simulink model "testVisualizer2023b"  (R2023b)
settings: Solver=FixedStepDiscrete  StartTime=time_s(1)  StopTime=time_s(end)  FixedStep=time_s(2) - time_s(1)  RelTol=1e-3
InitFcn:
  | loadParameters
libraries: dspnetwork x1
settings Model: Creator=MONSTER  LastModifiedBy=MONSTER
settings RTWCC: GPUComputeCapability=5.0

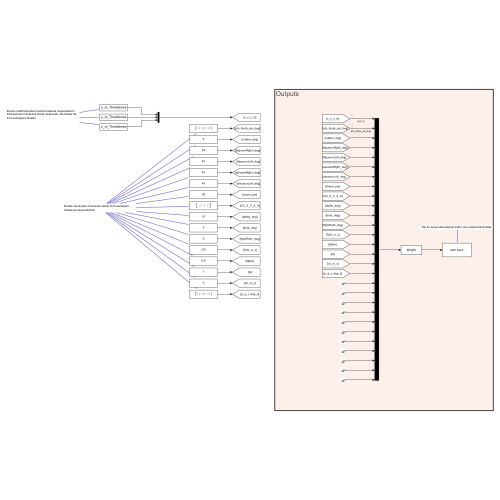
[thumbnail: Simulink's stored preview of the top-level diagram]
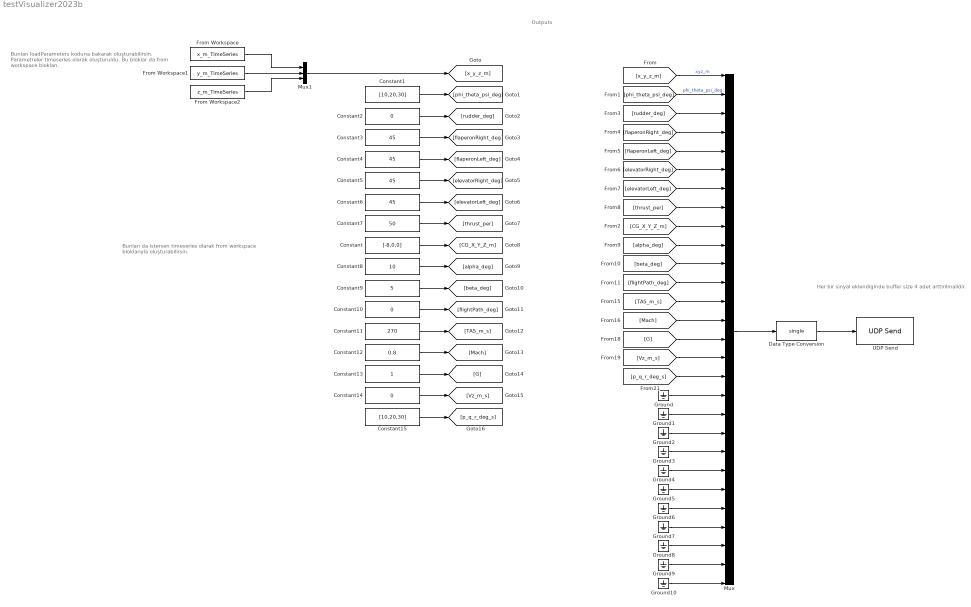
== system testVisualizer2023b ==
  note: Bunları loadParameters koduna bakarak oluşturabilirsin. Parametreler timeseries olarak oluşturuldu. Bu bloklar da from workspace blokları.
  note: Outputs
  note: Her bir sinyal eklendiginde buffer size 4 adet arttirilmalidir.
  note: Bunları da istersen timeseries olarak from workspace bloklarıyla oluşturabilirsin.
  Constant : Constant  Value=[-8,0,0]
  Constant1 : Constant  Value=[10,20,30]
  Constant10 : Constant  Value=0
  Constant11 : Constant  Value=270
  Constant12 : Constant  Value=0.8
  Constant13 : Constant
  Constant14 : Constant  Value=0
  Constant15 : Constant  Value=[10,20,30]
  Constant2 : Constant  Value=0
  Constant{3..6} (4 alike) : Constant  Value=45
  Constant7 : Constant  Value=50
  Constant8 : Constant  Value=10
  Constant9 : Constant  Value=5
  Data Type Conversion : DataTypeConversion  OutDataTypeStr=single  SaturateOnIntegerOverflow=off  RndMeth=Floor
  From Workspace : FromWorkspace  VariableName=x_m_TimeSeries
  From Workspace1 : FromWorkspace  VariableName=y_m_TimeSeries
  From Workspace2 : FromWorkspace  VariableName=z_m_TimeSeries
  Ground{,1..10} (11 alike) : Ground
  Mux : Mux  Inputs=28
  Mux1 : Mux  Inputs=3
  UDP Send : dspnetwork/UDP Send  remoteURL='127.0.0.1'  remotePort=8001  localURL='0.0.0.0'  localPortSource=Automatically determine  localPort=-1  sendBufferSize=29*4 + 107*4  sampletime=-1  blockPlatform=[]  separateLengthPort=0
  wires:
  Mux/1 -> Data Type Conversion/1
  Ground1/1 -> Mux/19
  Ground/1 -> Mux/18
  [beta_deg] -> Mux/11
  [p_q_r_deg_s] -> Mux/17
  [G] -> Mux/15
  [Mach] -> Mux/14
  [TAS_m_s] -> Mux/13
  [alpha_deg] -> Mux/10
  [x_y_z_m] -> Mux/1  "xyz_m"
  [flaperonLeft_deg] -> Mux/5
  [elevatorLeft_deg] -> Mux/7
  [phi_theta_psi_deg] -> Mux/2  "phi_theta_psi_deg"
  [flightPath_deg] -> Mux/12
  [thrust_per] -> Mux/8
  [CG_X_Y_Z_m] -> Mux/9
  [elevatorRight_deg] -> Mux/6
  [Vz_m_s] -> Mux/16
  Data Type Conversion/1 -> UDP Send/1
  [flaperonRight_deg] -> Mux/4
  [rudder_deg] -> Mux/3
  Constant/1 -> [CG_X_Y_Z_m]
  Ground2/1 -> Mux/20
  Ground3/1 -> Mux/21
  Ground5/1 -> Mux/23
  Ground4/1 -> Mux/22
  Ground6/1 -> Mux/24
  Ground7/1 -> Mux/25
  Ground9/1 -> Mux/27
  Ground8/1 -> Mux/26
  Ground10/1 -> Mux/28
  From Workspace2/1 -> Mux1/3
  From Workspace1/1 -> Mux1/2
  From Workspace/1 -> Mux1/1
  Mux1/1 -> [x_y_z_m]
  Constant1/1 -> [phi_theta_psi_deg]
  Constant2/1 -> [rudder_deg]
  Constant3/1 -> [flaperonRight_deg]
  Constant4/1 -> [flaperonLeft_deg]
  Constant5/1 -> [elevatorRight_deg]
  Constant6/1 -> [elevatorLeft_deg]
  Constant7/1 -> [thrust_per]
  Constant8/1 -> [alpha_deg]
  Constant9/1 -> [beta_deg]
  Constant10/1 -> [flightPath_deg]
  Constant11/1 -> [TAS_m_s]
  Constant12/1 -> [Mach]
  Constant13/1 -> [G]
  Constant14/1 -> [Vz_m_s]
  Constant15/1 -> [p_q_r_deg_s]
